simulink model "ZT_VehCtrl_18B"  (R2018b)
settings: Solver=FixedStepAuto  StartTime=0.0  StopTime=inf  FixedStep=0.005  RelTol=1e-3
InitFcn:
  | mbd_mpc_consistency_checks(bdroot(gcs));
undefined symbols (not defined in the file or in its folder): ANG_DEAD, BMS_NormalPwr, BrkPrsByBrkPct_TB_X, BrkPrsByBrkPct_TB_Y, DELAY_DISCHARGE, DELAY_RCUOFF, DRV_BACKWARD, DRV_BRAKE, DRV_FORWARD, DRV_NEUTRAL, DRV_PARK, DRV_UNPARK, DRV_ZEROTURN, EPB_LOCK, EPB_UNLOCK, ExtraLoadPwr, FanOff, fifo_0_vect, fifo_1_vect, HiFanReq, HV_finished, HV_No_Active, HV_POWER_OFF, HV_POWER_ON, HVDown, HVON, KaTLS_v_DrgUp_X_VehSpd, KeFTM_s_Way1OffDlyTime, KeFTM_TK_Way1CoolLv2OffBatTemp, KeFTM_TK_Way1CoolLv2OffMtrTemp, KeFTM_TK_Way1CoolLv2OnBatTemp, KeFTM_TK_Way1CoolLv2OnMtrTemp, KeFTM_TK_Way1CoolLv3OffBatTemp, KeFTM_TK_Way1CoolLv3OffMtrTemp, KeFTM_TK_Way1CoolLv3OnBatTemp, KeFTM_TK_Way1CoolLv3OnMtrTemp, KeFTM_TK_Way1CoolLv4OffBatTemp, KeFTM_TK_Way1CoolLv4OffMtrTemp, KeFTM_TK_Way1CoolLv4OnBatTemp, KeFTM_TK_Way1CoolLv4OnMtrTemp, Kp1, Kp2, LowFanReq, LQFP, MtrPwrFactor_RCU, MtrPwrHighToMidThd, MtrPwrLowToMidThd, MtrPwrMidToHighThd, MtrPwrMidToLowThd, MtrTrqMax, PCT_DEAD, Precharge, PTO_1000, PTO_540, pts1_fifo_0_vect, pts1_fifo_1_vect, pts2_fifo_0_vect, pts2_fifo_1_vect, pts3_fifo_0_vect, pts3_fifo_1_vect ... (+24)
libraries: mbd_mpc574x_ec_toolbox x173, canmsglib x72, simulink x57
(part 12 of 12)

== stateflow chart ZT_VehCtrl_18B/VehCtrl/MontionControl/ValveControl/BrakeSys/Chart ==
  state Decrease
    during:
    BrkValve = brakecontrol(BrkPrsTgt,BrkPrs);
  state ldle
    during:
    BrkValve = BrkValve;  % 保持不变
  state Increase
    during:
    BrkValve = brakecontrol(BrkPrsTgt,BrkPrs);
  (default) -> ldle
  ldle -> Decrease [order 1] : [BrkPrsTgt < BrkPrs - deadband]
  ldle -> Increase [order 2] : [BrkPrsTgt > BrkPrs + deadband]
  Increase -> ldle : [abs(BrkPrsTgt - BrkPrs) <= deadband]
  Decrease -> ldle : [abs(BrkPrsTgt - BrkPrs) <= deadband]
  data: brk_prstgt function_input; brk_prs function_input; breakvalue function_output; Ts function_input; deadband local double =10; BrkPrs input; BrkPrsTgt input; BrkValve output double
  function breakvalue = brakecontrol(brk_prstgt, brk_prs, Ts):
    | function breakvalue = brakecontrol(brk_prstgt, brk_prs, Ts)
    | % BRAKE_CONTROL_PID 刹车压力闭环PID控制函数 (Matlab 实现)
    | %
    | % 输入:
    | %   brk_prstgt: 期望刹车压力 (0-100%)
    | %   brk_prs:    当前实际刹车压力 (0-100%)
    | %   Ts:         控制周期时间 (秒), 例如 0.01s (10ms)
    | %
    | % 输出:
    | %   valve_output: 刹车阀输出指令 (0-2048, 整数)
    | 
    | % --- 1. 定义 PID 参数 ---
    | % 这些参数需要通过实际系统测试进行整定（Tuning）
    | Kp = 5.0;     % 比例增益 (通常是主导项)
    | Ki = 0.5;     % 积分增益 (消除稳态误差)
    | Kd = 0.01;    % 微分增益 (抑制超调)
    | Ts=0.005;
    | % --- 2. 硬件与比例定义 ---
    | VALVE_MAX = 2048.0;     % 阀门输出最大值
    | SCALE_FACTOR = VALVE_MAX / 100.0; % 比例因子 (2048 / 100 = 20.48)
    | 
    | % --- 3. 持久化状态 (用于积分项和微分项) ---
    | % 使用 persistent 关键字使变量在函数调用结束后仍保持其值
    | persistent integral_term prev_error
    | 
    | % 初始化持久化变量
    | if isempty(integral_term)
    |     integral_term = 0.0;
    |     prev_error = 0.0;
    | end
    | 
    | % --- 4. 核心 PID 计算 ---
    | 
    | % a. 计算误差
    | error = brk_prstgt - brk_prs;
    | 
    | % b. 比例项 (P Term)
    | P_out = Kp * error;
    | 
    | % c. 积分项 (I Term)
    | integral_term = integral_term + error * Ts;
    | 
    | % **防积分饱和 (Anti-windup)**: 限制积分项累积
    | % 限制范围：I_out 的绝对值不能超过 VALVE_MAX
    | integral_max = VALVE_MAX / Ki;
    | if integral_term > integral_max
    |     integral_term = integral_max;
    | elseif integral_term < 0
    |     % 刹车控制通常是单向的（只有压力增加），但为了通用性保留负限幅
    |     integral_term = max(integral_term, -integral_max); 
    | end
    | I_out = Ki * integral_term;
    | 
    | % d. 微分项 (D Term)
    | % 计算误差变化率 (微分)
    | derivative = (error - prev_error) / Ts;
    | D_out = Kd * derivative;
    | 
    | % --- 5. 总输出与限幅 ---
    | 
    | % e. 计算总控制信号 (百分比量纲)
    | control_signal_perc = P_out + I_out + D_out;
    | 
    | % f. 转换为硬件输出量程 (0-2048)
    | breakvalve_raw = control_signal_perc * SCALE_FACTOR;
    | 
    | % g. 硬件输出限幅 (Clamping)
    | if breakvalve_raw > VALVE_MAX
    |     breakvalve_raw = VALVE_MAX;
    | elseif breakvalve_raw < 0.0
    |     breakvalve_raw = 0.0;
    | end
    | 
    | % h. 更新状态
    | prev_error = error;
    | 
    | % --- 6. 返回结果 ---
    | breakvalue = round(breakvalve_raw); % 返回整数指令
    | end

== stateflow chart ZT_VehCtrl_18B/VehCtrl/FaultProc/Subsystem5/TimeOutLevel_RMT2 ==
  state on
    en:TimeOutLevel=1;LifeTemp=LiveCounter;
    du:LifeTemp=LiveCounter;
  state on_cnt
    en:TimeOutLevel=1;cnt=0;
    du:cnt = cnt + 1;
  state off
    en:TimeOutLevel=0;
  (default) -> on
  on -> on_cnt : [LiveCounter==LifeTemp]
  on_cnt -> on [order 2] : [LiveCounter~=LifeTemp]
  off -> on : [LiveCounter~=LifeTemp]
  on_cnt -> off [order 1] : [(cnt>=10)]
  data: LiveCounter input; TimeOutLevel output; LifeTemp local; cnt local

== stateflow chart ZT_VehCtrl_18B/VehCtrl/FaultProc/Subsystem5/PacketLoss_RMT2 ==
  state on
    en:PacketLossFlg=0;
  state on_cnt
    en:PacketLossFlg=0;cnt=0;
    du:cnt = cnt + 1;
  state off
    en:PacketLossFlg=1;
  (default) -> on
  on -> on_cnt : [(PacketLoss==1)||(CheckSum==1)]
  on_cnt -> on [order 2] : [(PacketLoss==0)&(CheckSum==0)]
  off -> on : [(PacketLoss==0)&(CheckSum==0)]
  on_cnt -> off [order 1] : [(cnt>=10)]
  data: CheckSum input; PacketLossFlg output; cnt local; PacketLoss input

== stateflow chart ZT_VehCtrl_18B/VehCtrl/EnergyManage1/Chart1 ==
  state Low
    during:
    RCU_RexGenPwr = RexGenPwrLow;
  state Mid
    during:
    RCU_RexGenPwr = RexGenPwrMid;
  state High
    during:
    RCU_RexGenPwr = RexGenPwrHigh;
  (default) -> Low
  Low -> Mid : [MtrPwrTotal >= MtrPwrLowToMidThd]
  Mid -> Low [order 1] : [MtrPwrTotal <= MtrPwrMidToLowThd]
  Mid -> High [order 2] : [MtrPwrTotal >= MtrPwrMidToHighThd]
  High -> Mid : [MtrPwrTotal <= MtrPwrHighToMidThd]
  data: MtrPwrHighToMidThd parameter; MtrPwrLowToMidThd parameter; MtrPwrMidToHighThd parameter; MtrPwrMidToLowThd parameter; MtrPwrTotal input; RCU_RexGenPwr output; RexGenPwrHigh parameter; RexGenPwrLow parameter; RexGenPwrMid parameter
